simulink model "noise_filter_for_velocities"  (R2022b)
settings: Solver=VariableStepAuto  StartTime=0.0  StopTime=10.0  RelTol=1e-3
libraries: simulink x1
settings Model: Creator=papaveneti  LastModifiedBy=papaveneti

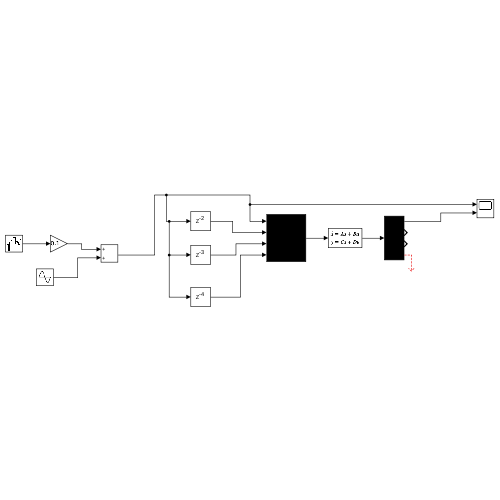
[thumbnail: Simulink's stored preview of the top-level diagram]
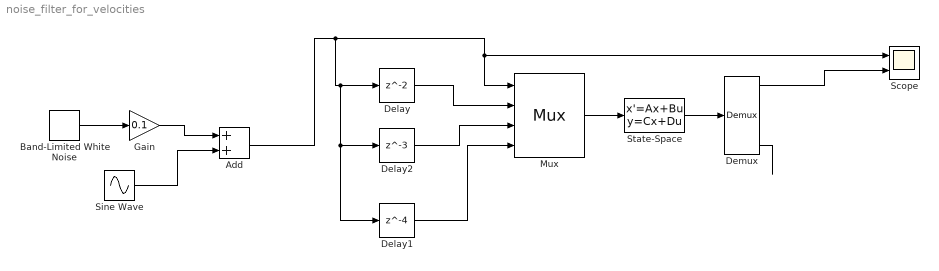
== system noise_filter_for_velocities ==
  Add : Sum
  Band-Limited White Noise : simulink/Sources/Band-Limited White Noise  Cov=[0.1]  Ts=0.01  seed=[23341]
  Delay : Delay
  Delay1 : Delay  DelayLength=4
  Delay2 : Delay  DelayLength=3
  Demux : Demux
  Gain : Gain  Gain=0.1
  Mux : Mux
  Scope : Scope  NumInputPorts=2
  Sine Wave : Sin  SampleTime=0
  State-Space : StateSpace  A=diag([-5,-5,-5,-5])  B=2*eye(4)  C=2.5*eye(4)  D=zeros(4,4)  InitialCondition=0
  wires:
  Band-Limited White Noise/1 -> Gain/1
  Delay/1 -> Mux/2
  Delay1/1 -> Mux/4
  Delay2/1 -> Mux/3
  Mux/1 -> State-Space/1
  State-Space/1 -> Demux/1
  Demux/4 -> ?
  Demux/1 -> Scope/2
  Gain/1 -> Add/1
  Sine Wave/1 -> Add/2
  Add/1 -> Delay1/1, Delay2/1, Delay/1, Scope/1, Mux/1
